simulink model "MPC"  (R2018a)
settings: Solver=ode1  StartTime=0.0  StopTime=inf  FixedStep=Td  RelTol=1e-3  EnableMultiTasking=on
values from neighbouring files (symbols this model uses):
  A_iq = [A_iq, -ones(size_A_iq(1), 1); zeros(1, size_A_iq(2)), -1]    [MPC_init.m]
  h_02 = h02    [MPC_init.m]
  L = repmat(eye(2),Nc,1)    [MPC_init.m]
  m = 2    [MPC_init.m]
  Nc = 2    [MPC_init.m]
  Np = 20    [MPC_init.m]
  Qy = 1*eye(1*Np)    [MPC_init.m]
  roh = 100    [MPC_init.m]
  Td = 0.5    [MPC_init.m]
  u_max = repmat(u_max,Nc,1)    [MPC_init.m]
  u_min = repmat(u_min,Nc,1)    [MPC_init.m]
  ue = [ue1; ue2]    [MPC_init.m]
  W_delta = [W_delta, zeros(size_W_delta(1), 1); zeros(1, size_W_delta(2)), 0]    [MPC_init.m]
  x_max = repmat(x_max,Np,1)    [MPC_init.m]
  x_min = repmat(x_min,Np,1)    [MPC_init.m]
  xe = [xe1; xe2]    [MPC_init.m]
  xe2 = 25.53    [MPC_init.m]
undefined symbols (not defined in the file or in its folder): Fx, Fy, gainh1, gainh2, Gx, Gy, h01, h02, HIL, Hy, offseth1, offseth2
libraries: simulink x3, quarc_library x3
settings Model: SimulationMode=external  Creator=steinbe  LastModifiedBy=local
settings SolverCC: PositivePriorityOrder=on
settings DataIOCC: SaveFormat=Array  SignalLoggingSaveFormat=ModelDataLogs
settings OptimizationCC: LifeSpan=inf
settings DebuggingCC: SFExecutionAtInitializationDiag=none
settings HardwareCC: ProdBitPerPointer=32  ProdBitPerSizeT=32  ProdBitPerPtrDiffT=32  ProdLargestAtomicFloat=None  ProdIntDivRoundTo=Undefined  ProdEndianess=Unspecified  ProdWordSize=32  ProdHWDeviceType=Generic->Unspecified (assume 32-bit Generic)
settings SFSimCC: SimCustomHeaderCode="#include \"qpOASES_wrapper_Simulink.h\""  SimUserLibraries=qpOasesLib.lib
settings SFSimCC: SimUserIncludeDirs=|
  | C:\Users\Public\Documents\qpOases\include
  | C:\Users\Public\Documents\qpOases\x64\Release
settings RTWCC: SystemTargetFile=quarc_win64.tlc  TemplateMakefile=quarc_default_tmf  Description=QUARC Win64 Target  RTWUseSimCustomCode=on  CustomHeaderCode="#include \"qpOASES_wrapper_Simulink.h\""  CustomLibrary=qpOasesLib.lib
settings RTWCC: CustomInclude=|
  | C:\Users\Public\Documents\qpOases\include
  | C:\Users\Public\Documents\qpOases\x64\Release
settings CodeAppCC: StateflowObjectComments=on
settings STFCustomTargetCC: TargetPreCompLibLocation=C:\PROGRA~3\QUARC\lib\2018a\win64\release  ConcurrentExecutionCompliant=on  GeneratePreprocessorConditionals=Disable all  SystemTargetFile=quarc_win64.tlc
settings GRTTargetCC: TargetPreCompLibLocation=C:\PROGRA~3\QUARC\lib\2018a\win64\release  TargetLangStandard=C89/C90 (ANSI)  ParMdlRefBuildCompliant=off  CompOptLevelCompliant=off  GeneratePreprocessorConditionals=Disable all  CombineOutputUpdateFcns=off  MatFileLogging=off  CPPClassGenCompliant=off  GRTInterface=on  UseToolchainInfoCompliant=off  ExtMode=on  ExtModeMexFile=quarc_comm

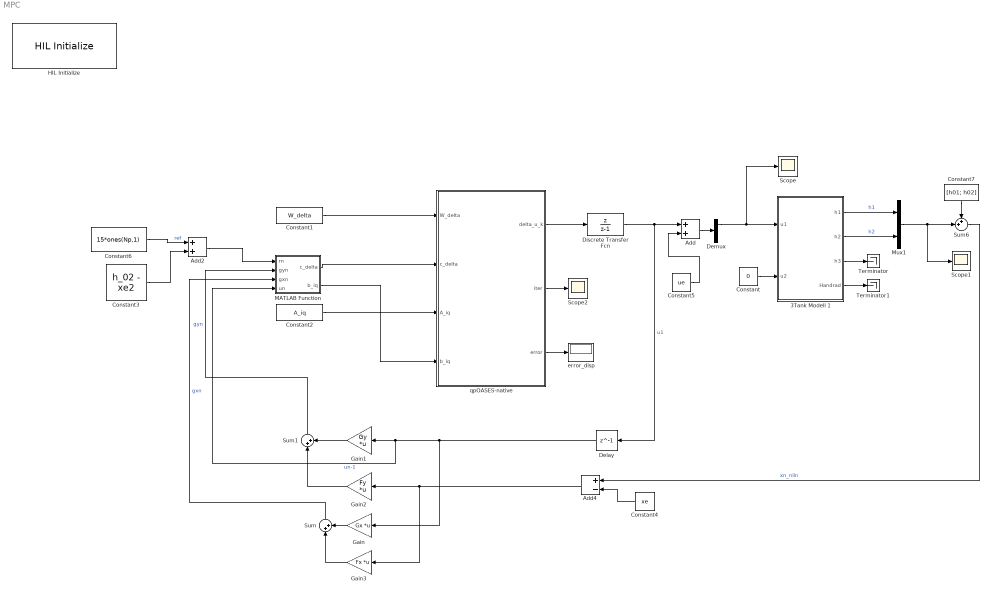
== system MPC ==
  3Tank Modell 1 : Subsystem
  Add : Sum
  Add2 : Sum
  Add4 : Sum  Inputs=+-
  Constant : Constant  Value=0
  Constant1 : Constant  Value=W_delta
  Constant2 : Constant  Value=A_iq
  Constant3 : Constant  Value=h_02 - xe2
  Constant4 : Constant  Value=xe
  Constant5 : Constant  Value=ue
  Constant6 : Constant  Value=15*ones(Np,1)
  Constant7 : Constant  Value=[h01; h02]
  Delay : Delay  DelayLength=1  InitialCondition=[0;0]  SampleTime=Td
  Demux : Demux  Outputs=2
  Discrete Transfer Fcn : DiscreteTransferFcn  Numerator=[1 0]  Denominator=[1 -1]  InitialStates=[0;0]  SampleTime=Td
  Gain : Gain  Gain=Gx  Multiplication=Matrix(K*u)
  Gain1 : Gain  Gain=Gy  Multiplication=Matrix(K*u)
  Gain2 : Gain  Gain=Fy  Multiplication=Matrix(K*u)
  Gain3 : Gain  Gain=Fx  Multiplication=Matrix(K*u)
  HIL Initialize : quarc_library/Data Acquisition/Generic/Configuration/HIL Initialize  object_name=HIL-1  board_type=q8_usb  board_number=0  board_options=update_rate=normal;decimation=1  exclusive=off  active=on  hardware_clocks=[0:2]  clock_modes=[]  initial_clock_frequencies=[]  set_clock_params_at_start=off  set_clock_params_at_switch_in=off  set_clock_frequencies_at_start=off  set_clock_frequencies_at_switch_in=off  analog_input_channels=[0:7]  analog_input_configurations=[]  analog_input_maximums=10  analog_input_minimums=-10  set_analog_input_params_at_start=on  set_analog_input_params_at_switch_in=off  analog_output_channels=[0:7]  analog_output_maximums=10  analog_output_minimums=-10  initial_analog_outputs=[0]  final_analog_outputs=[0]  watchdog_analog_outputs=0  set_analog_output_params_at_start=on  set_analog_output_params_at_switch_in=off  set_analog_outputs_at_start=on  set_analog_outputs_at_switch_in=off  set_analog_outputs_at_terminate=on  set_analog_outputs_at_switch_out=off  set_analog_outputs_on_watchdog=off  digital_input_channels=[]  digital_output_channels=[]  digital_output_configuration=[]  initial_digital_outputs=[1]  final_digital_outputs=[1]  watchdog_digital_outputs=[1]  set_digital_output_params_at_start=off  set_digital_output_params_at_switch_in=off  set_digital_outputs_at_start=on  set_digital_outputs_at_switch_in=off  set_digital_outputs_at_terminate=on  set_digital_outputs_at_switch_out=off  set_digital_outputs_on_watchdog=off  encoder_channels=[0:7]  quadrature=[4]  encoder_filter_frequency=[]  initial_encoder_counts=[0]  set_encoder_params_at_start=on  set_encoder_params_at_switch_in=off  set_encoder_counts_at_start=on  set_encoder_counts_at_switch_in=off  pwm_channels=[0:7]  pwm_modes=0  pwm_frequency=99.532799999999995e6/4095  pwm_configuration=[0]  pwm_alignment=[0]  pwm_polarity=[1]  pwm_leading_deadband=[0]  pwm_trailing_deadband=[0]  initial_pwm_outputs=[0]  final_pwm_outputs=[0]  watchdog_pwm_outputs=[0]  set_pwm_params_at_start=on  set_pwm_params_at_switch_in=off  set_pwm_outputs_at_start=on  set_pwm_outputs_at_switch_in=off  set_pwm_outputs_at_terminate=on  set_pwm_outputs_at_switch_out=off  set_pwm_outputs_on_watchdog=off  other_output_channels=[]  initial_other_outputs=[]  final_other_outputs=[]  watchdog_other_outputs=[]  set_other_outputs_at_start=off  set_other_outputs_at_switch_in=off  set_other_outputs_at_terminate=off  set_other_outputs_at_switch_out=off  set_other_outputs_on_watchdog=off
  MATLAB Function : MATLAB Function  TreatAsAtomicUnit=on
  Mux1 : Mux  Inputs=2
  Scope : Scope
  Scope1 : Scope
  Scope2 : Scope
  Sum : Sum  Inputs=|++
  Sum1 : Sum  Inputs=|++
  Sum6 : Sum  Inputs=++|
  Terminator : Terminator
  Terminator1 : Terminator
  error_disp : Display
  qpOASES-native : MATLAB Function  TreatAsAtomicUnit=on
  wires:
  qpOASES-native/1(delta_u_k) -> Discrete Transfer Fcn/1
  Discrete Transfer Fcn/1 -> Add/1, Delay/1  "u1"
  3Tank Modell 1/1(h1) -> Mux1/1  "h1"
  3Tank Modell 1/2(h2) -> Mux1/2  "h2"
  Constant7/1 -> Sum6/1
  Mux1/1 -> Sum6/2, Scope1/1
  3Tank Modell 1/3(h3) -> Terminator/1
  3Tank Modell 1/4(Handrad) -> Terminator1/1
  qpOASES-native/2(iter) -> Scope2/1
  qpOASES-native/3(error) -> error_disp/1
  Constant/1 -> 3Tank Modell 1/2(u2)
  MATLAB Function/1(c_delta) -> qpOASES-native/2(c_delta)
  Constant1/1 -> qpOASES-native/1(W_delta)
  Constant2/1 -> qpOASES-native/3(A_iq)
  MATLAB Function/2(b_iq) -> qpOASES-native/4(b_iq)
  Constant6/1 -> Add2/1  "ref"
  Constant3/1 -> Add2/2
  Add2/1 -> MATLAB Function/1(rn)
  Delay/1 -> Gain/1, MATLAB Function/4(un), Gain1/1  "un-1"
  Gain2/1 -> Sum1/1
  Sum1/1 -> MATLAB Function/2(gyn)  "gyn"
  Sum/1 -> MATLAB Function/3(gxn)  "gxn"
  Gain3/1 -> Sum/1
  Add4/1 -> Gain3/1, Gain2/1
  Gain/1 -> Sum/2
  Gain1/1 -> Sum1/2
  Constant4/1 -> Add4/2
  Sum6/1 -> Add4/1  "xn_nlin"
  Demux/1 -> Scope/1, 3Tank Modell 1/1(u1)
  Constant5/1 -> Add/2
  Add/1 -> Demux/1

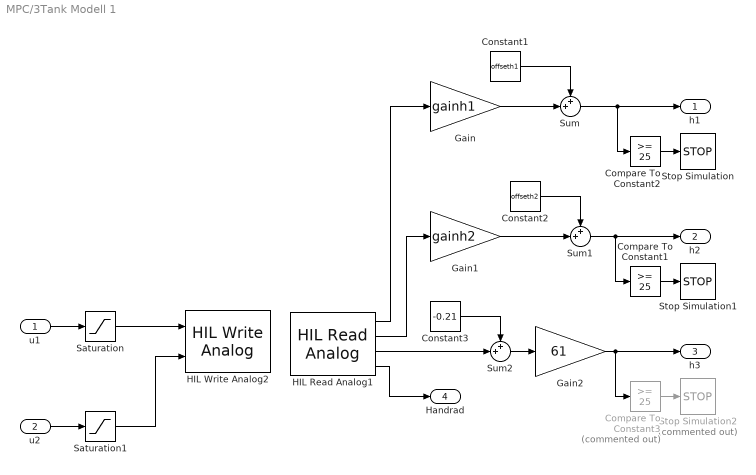
== system MPC/3Tank Modell 1 ==
  u1 : Inport
  u2 : Inport  Port=2
  Compare To Constant1 : simulink/Logic and Bit Operations/Compare To Constant  relop=>=  const=25  OutDataTypeStr=boolean  ZeroCross=off
  Compare To Constant2 : simulink/Logic and Bit Operations/Compare To Constant  relop=>=  const=25  OutDataTypeStr=boolean  ZeroCross=off
  Compare To Constant3 : simulink/Logic and Bit Operations/Compare To Constant  Commented=on  relop=>=  const=25  OutDataTypeStr=boolean  ZeroCross=off
  Constant1 : Constant  Value=offseth1
  Constant2 : Constant  Value=offseth2
  Constant3 : Constant  Value=-0.21
  Gain : Gain  Gain=gainh1
  Gain1 : Gain  Gain=gainh2
  Gain2 : Gain  Gain=61
  HIL Read Analog1 : quarc_library/Data Acquisition/Generic/Immediate I//O/HIL Read Analog  object_name=HIL-1  channels=[0:3]  sample_time=qc_get_step_size  active=on  vector_output=off
  HIL Write Analog2 : quarc_library/Data Acquisition/Generic/Immediate I//O/HIL Write Analog  object_name=HIL-1  channels=[0:1]  sample_time=-1  active=off  vector_input=off
  Saturation : Saturate  UpperLimit=10  LowerLimit=0
  Saturation1 : Saturate  UpperLimit=10  LowerLimit=0
  Stop Simulation : Stop
  Stop Simulation1 : Stop
  Stop Simulation2 : Stop  Commented=on
  Sum : Sum  Inputs=++|
  Sum1 : Sum  Inputs=++|
  Sum2 : Sum  Inputs=++|
  h1 : Outport
  h2 : Outport  Port=2
  h3 : Outport  Port=3
  Handrad : Outport  Port=4
  wires:
  u1/1 -> Saturation/1
  u2/1 -> Saturation1/1
  Saturation/1 -> HIL Write Analog2/1
  Saturation1/1 -> HIL Write Analog2/2
  HIL Read Analog1/4 -> Handrad/1
  Compare To Constant2/1 -> Stop Simulation/1
  Compare To Constant1/1 -> Stop Simulation1/1
  Gain2/1 -> Compare To Constant3/1, h3/1
  Compare To Constant3/1 -> Stop Simulation2/1
  Sum1/1 -> Compare To Constant1/1, h2/1
  Sum/1 -> h1/1, Compare To Constant2/1
  HIL Read Analog1/1 -> Gain/1
  Constant1/1 -> Sum/1
  Constant2/1 -> Sum1/1
  HIL Read Analog1/2 -> Gain1/1
  Constant3/1 -> Sum2/1
  Sum2/1 -> Gain2/1
  HIL Read Analog1/3 -> Sum2/2
  Gain/1 -> Sum/2
  Gain1/1 -> Sum1/2

== matlab function MPC/MATLAB Function ==
  data: rn input; c_delta output; gyn input; gxn input; b_iq output; un input; Qy parameter; L parameter; u_min parameter; u_max parameter; x_min parameter; x_max parameter; Hy parameter; roh parameter
function [c_delta, b_iq] = fcn(rn, gyn, gxn, un, Qy, L, u_min, u_max, x_min, x_max, Hy, roh)
w_bar = [L*un-u_min;u_max-L*un;gxn-x_min;x_max-gxn];
en = gyn - rn;
c_delta = [2'*Hy'*Qy*en; roh];
b_iq = [w_bar; roh];

== matlab function MPC/qpOASES-native ==
  data: W_delta input; delta_u_k output; c_delta input; A_iq input; b_iq input; iter output; error output; m parameter; Nc parameter
function [delta_u_k, iter, error] = fcn(W_delta, c_delta, A_iq, b_iq, m, Nc)
    
    persistent initialized options;
    % qpOASES uses row-major matrix storage (Matlab: column-major)!!!
    A_iq_tr = A_iq';
    
    delta_u_hat_k = coder.nullcopy(zeros(m * Nc, 1));
    lambda = coder.nullcopy(zeros(size(W_delta, 1) + size(A_iq, 1), 1));
    J = coder.nullcopy(double(0));
    iter = int32(180);
    
    if (isempty(initialized))
        options = coder.opaque('qpOASES_Options', 'HeaderFile', 'qpOASES_wrapper_Simulink.h');
        coder.ceval('qpOASES_Options_init', coder.wref(options), int32(2));
        coder.ceval('QProblem_setup', int32(size(W_delta, 1)), int32(size(A_iq, 1)), int32(6));
        
        initialized = 1;
    end
    
    error = coder.nullcopy(int32(0));
    coder.ceval('QProblem_init', coder.rref(W_delta), coder.rref(c_delta), ...
        coder.rref(A_iq_tr), [], [], [], coder.rref(b_iq), coder.ref(iter), ...
        [], coder.rref(options), coder.ref(delta_u_hat_k), coder.ref(lambda), ...
        coder.ref(J), coder.ref(error)); 
    
    delta_u_k = delta_u_hat_k(1 : m);
    
%     coder.ceval('QProblem_cleanup');
end
